simulink model "parcours_funktioniert"  (R2018a)
settings: Solver=ode1  StartTime=0.0  StopTime=inf  FixedStep=1/20  RelTol=1e-3  EnableMultiTasking=on
undefined symbols (not defined in the file): gray
libraries: simulink x6, visiontextngfix x4, visiontransforms x4, visionanalysis x2, visionstatistics x2, PiCar_library x1, embdlinuxlib x1
settings Model: SimulationMode=external  Creator=raspberry  LastModifiedBy=dave
settings SolverCC: PositivePriorityOrder=on
settings OptimizationCC: PassReuseOutputArgsAs=Individual arguments  MaxStackSize=64
settings DebuggingCC: ParameterTunabilityLossMsg=error
settings HardwareCC: ProdBitPerPointer=32  ProdBitPerSizeT=32  ProdBitPerPtrDiffT=32  ProdLargestAtomicInteger=Long  ProdLargestAtomicFloat=Double  ProdWordSize=32  ProdHWDeviceType=ARM Compatible->ARM Cortex
settings SFSimCC: MATLABDynamicMemAlloc=off
settings RTWCC: SystemTargetFile=ert.tlc  HardwareBoard=Raspberry Pi  TLCOptions="-aInlineSetEventsForThisBaseRateFcn=TLC_FALSE -aSuppressMultiTaskScheduler=TLC_FALSE  -aRateBasedStepFcn=0"  TemplateMakefile=ert_default_tmf  Toolchain=GNU GCC Raspberry Pi
settings RTWCC: CustomTerminator=|
  | /* Send ALL_LED_OFF Signal to all PWM driver chip address
  | See PCA9685 user manual, section 7.3.4
  | Set Chip in sleep mode, section 7.3.1
  | Reset the PWM ON/OFF states for all LEDs */
  | 
  | int fd;
  | 
  | fd = wiringPiI2CSetup(0x70);
  | wiringPiI2CWriteReg8(fd, 0x00, 0x11); // sleep mode
  | wiringPiI2CWriteReg8(fd, 0xFD, 0x10); // all LED off
  | wiringPiI2CWriteReg8(fd, 0xFC, 0x00);
  | wiringPiI2CWriteReg8(fd, 0xFB, 0x00);
  | wiringPiI2CWriteReg8(fd, 0xFA, 0x00);
settings CodeAppCC: ForceParamTrailComments=on  IgnoreCustomStorageClasses=off  OperatorAnnotations=on  SimulinkDataObjDesc=on  SFDataObjDesc=on  MATLABFcnDesc=on  InsertBlockDesc=on  StateflowObjectComments=on  MATLABSourceComments=on
settings ERTTargetCC: SupportVariableSizeSignals=on

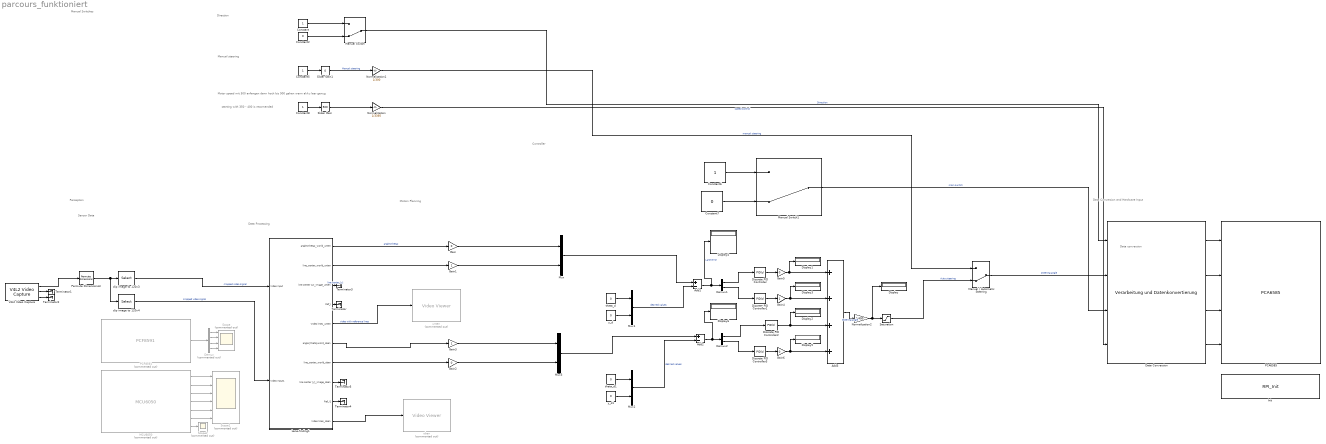
== system parcours_funktioniert ==
  note: starting with 350 - 400 is recomended
  note: Data Conversion and Hardware Input
  note: Data conversion
  note: Manual Switches
  note: Motion Planning
  note: Perception
  note: Controller
  note: Data Processing
  note: Sensor Data
  note: Manual steering
  note: Motor speed
      | mit 500 anfangen
      | dann hoch bis 900
      | gehen wenn akku
      | leer genug
  note: Direction
  Add1 : Sum  Inputs=+-
  Add2 : Sum  Inputs=+-
  Add3 : Sum  Inputs=++++
  Constant{,5..6,8} (4 alike) : Constant
  Constant2 : Constant  Value=0
  Constant7 : Constant  Value=0
  Data Conversion : PiCar_library/Verarbeitung und Datenkonvertierung
      link override Constant3: Value=1160
  Demux : Demux  Commented=on
  Demux1 : Demux  Outputs=2
  Demux2 : Demux  Outputs=2
  Discrete PID Controller : simulink/Continuous/PID Controller  Controller=PID  TimeDomain=Discrete-time  SampleTime=-1  IntegratorMethod=Forward Euler  FilterMethod=Forward Euler  Form=Parallel  UseFilter=on  ControllerParametersSource=internal  P=0  I=0  D=0  N=100  InitialConditionSource=internal  InitialConditionForIntegrator=0  InitialConditionForFilter=0  ExternalReset=none  LimitOutput=off  UpperSaturationLimit=inf  LowerSaturationLimit=-inf  LinearizeAsGain=off  AntiWindupMode=none  Kb=1  TrackingMode=off  Kt=1  PParamMin=[]  PParamMax=[]  IParamMin=[]  IParamMax=[]  DParamMin=[]  DParamMax=[]  NParamMin=[]  NParamMax=[]  KbParamMin=[]  KbParamMax=[]  KtParamMin=[]  KtParamMax=[]  POutMin=[]  POutMax=[]  IOutMin=[]  IOutMax=[]  DOutMin=[]  DOutMax=[]  NOutMin=[]  NOutMax=[]  KbOutMin=[]  KbOutMax=[]  KtOutMin=[]  KtOutMax=[]  IntegratorOutMin=[]  IntegratorOutMax=[]  FilterOutMin=[]  FilterOutMax=[]  SumOutMin=[]  SumOutMax=[]  SumI1OutMin=[]  SumI1OutMax=[]  SumI2OutMin=[]  SumI2OutMax=[]  SumI3OutMin=[]  SumI3OutMax=[]  SumDOutMin=[]  SumDOutMax=[]  SaturationOutMin=[]  SaturationOutMax=[]  IntegratorContinuousStateAttributes=''  IntegratorStateMustResolveToSignalObject=off  IntegratorRTWStateStorageClass=Auto  FilterContinuousStateAttributes=''  FilterStateMustResolveToSignalObject=off  FilterRTWStateStorageClass=Auto  DifferentiatorICPrevScaledInput=0  DifferentiatorOutMin=[]  DifferentiatorOutMax=[]  FilterDiffOutCoefMin=[]  FilterDiffOutCoefMax=[]  SumDenOutMin=[]  SumDenOutMax=[]  SumNumOutMin=[]  SumNumOutMax=[]  ReciprocalOutMin=[]  ReciprocalOutMax=[]  DivideOutMin=[]  DivideOutMax=[]  TunerSelectOption=Transfer Function Based (PID Tuner App)
  Discrete PID Controller1 : simulink/Continuous/PID Controller  Controller=PID  TimeDomain=Discrete-time  SampleTime=-1  IntegratorMethod=Forward Euler  FilterMethod=Forward Euler  Form=Parallel  UseFilter=on  ControllerParametersSource=internal  P=1  I=0  D=0  N=100  InitialConditionSource=internal  InitialConditionForIntegrator=0  InitialConditionForFilter=0  ExternalReset=none  LimitOutput=off  UpperSaturationLimit=inf  LowerSaturationLimit=-inf  LinearizeAsGain=off  AntiWindupMode=none  Kb=1  TrackingMode=off  Kt=1  PParamMin=[]  PParamMax=[]  IParamMin=[]  IParamMax=[]  DParamMin=[]  DParamMax=[]  NParamMin=[]  NParamMax=[]  KbParamMin=[]  KbParamMax=[]  KtParamMin=[]  KtParamMax=[]  POutMin=[]  POutMax=[]  IOutMin=[]  IOutMax=[]  DOutMin=[]  DOutMax=[]  NOutMin=[]  NOutMax=[]  KbOutMin=[]  KbOutMax=[]  KtOutMin=[]  KtOutMax=[]  IntegratorOutMin=[]  IntegratorOutMax=[]  FilterOutMin=[]  FilterOutMax=[]  SumOutMin=[]  SumOutMax=[]  SumI1OutMin=[]  SumI1OutMax=[]  SumI2OutMin=[]  SumI2OutMax=[]  SumI3OutMin=[]  SumI3OutMax=[]  SumDOutMin=[]  SumDOutMax=[]  SaturationOutMin=[]  SaturationOutMax=[]  IntegratorContinuousStateAttributes=''  IntegratorStateMustResolveToSignalObject=off  IntegratorRTWStateStorageClass=Auto  FilterContinuousStateAttributes=''  FilterStateMustResolveToSignalObject=off  FilterRTWStateStorageClass=Auto  DifferentiatorICPrevScaledInput=0  DifferentiatorOutMin=[]  DifferentiatorOutMax=[]  FilterDiffOutCoefMin=[]  FilterDiffOutCoefMax=[]  SumDenOutMin=[]  SumDenOutMax=[]  SumNumOutMin=[]  SumNumOutMax=[]  ReciprocalOutMin=[]  ReciprocalOutMax=[]  DivideOutMin=[]  DivideOutMax=[]  TunerSelectOption=Transfer Function Based (PID Tuner App)
  Discrete PID Controller2 : simulink/Continuous/PID Controller  Controller=PID  TimeDomain=Discrete-time  SampleTime=-1  IntegratorMethod=Forward Euler  FilterMethod=Forward Euler  Form=Parallel  UseFilter=on  ControllerParametersSource=internal  P=10  I=0  D=0  N=100  InitialConditionSource=internal  InitialConditionForIntegrator=0  InitialConditionForFilter=0  ExternalReset=none  LimitOutput=off  UpperSaturationLimit=inf  LowerSaturationLimit=-inf  LinearizeAsGain=off  AntiWindupMode=none  Kb=1  TrackingMode=off  Kt=1  PParamMin=[]  PParamMax=[]  IParamMin=[]  IParamMax=[]  DParamMin=[]  DParamMax=[]  NParamMin=[]  NParamMax=[]  KbParamMin=[]  KbParamMax=[]  KtParamMin=[]  KtParamMax=[]  POutMin=[]  POutMax=[]  IOutMin=[]  IOutMax=[]  DOutMin=[]  DOutMax=[]  NOutMin=[]  NOutMax=[]  KbOutMin=[]  KbOutMax=[]  KtOutMin=[]  KtOutMax=[]  IntegratorOutMin=[]  IntegratorOutMax=[]  FilterOutMin=[]  FilterOutMax=[]  SumOutMin=[]  SumOutMax=[]  SumI1OutMin=[]  SumI1OutMax=[]  SumI2OutMin=[]  SumI2OutMax=[]  SumI3OutMin=[]  SumI3OutMax=[]  SumDOutMin=[]  SumDOutMax=[]  SaturationOutMin=[]  SaturationOutMax=[]  IntegratorContinuousStateAttributes=''  IntegratorStateMustResolveToSignalObject=off  IntegratorRTWStateStorageClass=Auto  FilterContinuousStateAttributes=''  FilterStateMustResolveToSignalObject=off  FilterRTWStateStorageClass=Auto  DifferentiatorICPrevScaledInput=0  DifferentiatorOutMin=[]  DifferentiatorOutMax=[]  FilterDiffOutCoefMin=[]  FilterDiffOutCoefMax=[]  SumDenOutMin=[]  SumDenOutMax=[]  SumNumOutMin=[]  SumNumOutMax=[]  ReciprocalOutMin=[]  ReciprocalOutMax=[]  DivideOutMin=[]  DivideOutMax=[]  TunerSelectOption=Transfer Function Based (PID Tuner App)
  Discrete PID Controller3 : simulink/Continuous/PID Controller  Controller=PID  TimeDomain=Discrete-time  SampleTime=-1  IntegratorMethod=Forward Euler  FilterMethod=Forward Euler  Form=Parallel  UseFilter=on  ControllerParametersSource=internal  P=0  I=0  D=0  N=100  InitialConditionSource=internal  InitialConditionForIntegrator=0  InitialConditionForFilter=0  ExternalReset=none  LimitOutput=off  UpperSaturationLimit=inf  LowerSaturationLimit=-inf  LinearizeAsGain=off  AntiWindupMode=none  Kb=1  TrackingMode=off  Kt=1  PParamMin=[]  PParamMax=[]  IParamMin=[]  IParamMax=[]  DParamMin=[]  DParamMax=[]  NParamMin=[]  NParamMax=[]  KbParamMin=[]  KbParamMax=[]  KtParamMin=[]  KtParamMax=[]  POutMin=[]  POutMax=[]  IOutMin=[]  IOutMax=[]  DOutMin=[]  DOutMax=[]  NOutMin=[]  NOutMax=[]  KbOutMin=[]  KbOutMax=[]  KtOutMin=[]  KtOutMax=[]  IntegratorOutMin=[]  IntegratorOutMax=[]  FilterOutMin=[]  FilterOutMax=[]  SumOutMin=[]  SumOutMax=[]  SumI1OutMin=[]  SumI1OutMax=[]  SumI2OutMin=[]  SumI2OutMax=[]  SumI3OutMin=[]  SumI3OutMax=[]  SumDOutMin=[]  SumDOutMax=[]  SaturationOutMin=[]  SaturationOutMax=[]  IntegratorContinuousStateAttributes=''  IntegratorStateMustResolveToSignalObject=off  IntegratorRTWStateStorageClass=Auto  FilterContinuousStateAttributes=''  FilterStateMustResolveToSignalObject=off  FilterRTWStateStorageClass=Auto  DifferentiatorICPrevScaledInput=0  DifferentiatorOutMin=[]  DifferentiatorOutMax=[]  FilterDiffOutCoefMin=[]  FilterDiffOutCoefMax=[]  SumDenOutMin=[]  SumDenOutMax=[]  SumNumOutMin=[]  SumNumOutMax=[]  ReciprocalOutMin=[]  ReciprocalOutMax=[]  DivideOutMin=[]  DivideOutMax=[]  TunerSelectOption=Transfer Function Based (PID Tuner App)
  Display{,1..6} (7 alike) : Display
  Gain{,2,5..6} (4 alike) : Gain  Gain=0
  Gain1 : Gain
  Gain3 : Gain
  Gain4 : Gain
  Init : S-Function  Priority=1  InitFcn=try, set_param(gcb,'FunctionName','RPI_Init'), end  FunctionName=RPI_Init  SFunctionModules=RPI_Init_wrapper  SFunctionDeploymentMode=off  EnableBusSupport=off  mask(S-Function Builder){}
      mask help: Simulink:masks:SFunctionBuilder_MD
      mask init:
      | val = [[.9  0.75 0.75 1 1 .9 .9 1]',[1 1 0.75 0.75 .9 .9 1 .9]'];try , sys = get_param(gcb,'SfunBuilderFcnName');if isempty(sys), sys = get_param(gcb,'FunctionName'); end,catch, sys = get_param(gcb,'FunctionName'); end
      settings: CopyFcn=set_param(gcbh,'LinkStatus','none')  PreSaveFcn=try, set_param(gcb,'FunctionName','RPI_Init'), end  OpenFcn=sfunctionwizard(gcbh)
      mask Display:
      | plot(val(:,1),val(:,2))
      | disp(sys)
  Lane-finding1 : Subsystem  AncestorBlock=PiCar_library/Lane-finding
  MCU6050 : S-Function  Commented=on  InitFcn=try, set_param(gcb,'FunctionName','MCU6050'), end  FunctionName=MCU6050  SFunctionModules=MCU6050_wrapper  SFunctionDeploymentMode=off  EnableBusSupport=off  mask(S-Function Builder){}
      mask help: Simulink:masks:SFunctionBuilder_MD
      mask init: same as parcours_funktioniert/Init
      settings: CopyFcn=set_param(gcbh,'LinkStatus','none')  PreSaveFcn=try, set_param(gcb,'FunctionName','MCU6050'), end  OpenFcn=sfunctionwizard(gcbh)
      mask Display: plot(val(:,1),val(:,2)),disp(sys), port_label('output',1,'ax'), port_label('output',2,'ay'), port_label('output',3,'az'), port_label('output',4,'omx'), port_label('output',5,'omy'), port_label('output',6,'omz'), port_label('output',7,'temp')
  Manual / Automatic Steering : ManualSwitch  CurrentSetting=0
  Manual Switch : ManualSwitch  CurrentSetting=0
  Manual Switch1 : ManualSwitch  CurrentSetting=0
  Mux{,1..3} (4 alike) : Mux  Inputs=2
  Normalization : Gain  Gain=1/3395
  Normalization1 : Gain  Gain=1/300
  Normalization2 : Gain  Gain=1/400
  PCA6585 : S-Function  InitFcn=try, set_param(gcb,'FunctionName','PCA6585'), end  FunctionName=PCA6585  SFunctionModules=PCA6585_wrapper  SFunctionDeploymentMode=off  EnableBusSupport=off  mask(S-Function Builder){}
      mask help: Simulink:masks:SFunctionBuilder_MD
      mask init: same as parcours_funktioniert/Init
      settings: CopyFcn=set_param(gcbh,'LinkStatus','none')  PreSaveFcn=try, set_param(gcb,'FunctionName','PCA6585'), end  OpenFcn=sfunctionwizard(gcbh)
      mask Display: plot(val(:,1),val(:,2)),disp(sys), port_label('input',1,'IN_1'), port_label('input',2,'IN_2'), port_label('input',3,'PWM'), port_label('input',4,'SERVO')
  PCF8591 : S-Function  Commented=on  InitFcn=try, set_param(gcb,'FunctionName','PCF8591'), end  FunctionName=PCF8591  SFunctionModules=PCF8591_wrapper  SFunctionDeploymentMode=off  EnableBusSupport=off  mask(S-Function Builder){}
      mask help: Simulink:masks:SFunctionBuilder_MD
      mask init: same as parcours_funktioniert/Init
      settings: CopyFcn=set_param(gcbh,'LinkStatus','none')  PreSaveFcn=try, set_param(gcb,'FunctionName','PCF8591'), end  OpenFcn=sfunctionwizard(gcbh)
      mask Display: plot(val(:,1),val(:,2)),disp(sys), port_label('output',1,'PCF8591_out')
  Permute Dimensions3 : PermuteDimensions
  Saturation : Saturate  UpperLimit=1  LowerLimit=-1
  Scope : Scope  Commented=on  NumInputPorts=4
  Scope1 : Scope  Commented=on  NumInputPorts=6
  Scope2 : Scope  Commented=on
  Slider Gain : simulink/Math Operations/Slider Gain  gain=500  low=0  high=3395
  Slider Gain1 : simulink/Math Operations/Slider Gain  gain=0  low=-300  high=300
  Terminator{,1..5} (6 alike) : Terminator
  V4L2 Video Capture : embdlinuxlib/V4L2 Video Capture  m_devName='/dev/video0'  roi=[0, 0, 640, 480]  imSizeSelection=320x240  imSize=[640, 480]  pixelFormat=YCbCr 4:2:2  pixelOrder=Planar  sampleTime=1/20  simOutput=Colorbars  blockPlatform=Raspberry Pi
      settings: SourceProductName=Simulink Support Package for Raspberry Pi Hardware  SourceProductBaseCode=RASPPI
  clip image to 120x3 : Selector  NumberOfDimensions=2  InputPortWidth=3  IndexOptions=Index vector (dialog),Index vector (dialog)  Indices=[180:1:200],[1:4:320]  OutputSizes=1,1
  clip image to 120x4 : Selector  NumberOfDimensions=2  InputPortWidth=3  IndexOptions=Index vector (dialog),Index vector (dialog)  Indices=[120:1:180],[1:4:320]  OutputSizes=1,1
  oben : VideoViewer  Commented=on  colormapValue=gray(256)  FigPos=[37.8 442.8 582.4 304.8]
  theta_d : Constant  Value=0
  theta_d1 : Constant  Value=0
  unten : VideoViewer  Commented=on  colormapValue=gray(256)  FigPos=[19.4 847.6 603.2 284.8]
  y_d : Constant  Value=0
  y_d1 : Constant  Value=0
  wires:
  Constant/1 -> Manual Switch/1
  Constant2/1 -> Manual Switch/2
  Constant7/1 -> Manual Switch1/2
  Constant6/1 -> Manual Switch1/1
  Constant8/1 -> Slider Gain/1
  Slider Gain1/1 -> Normalization1/1  "Manual steering"
  Constant5/1 -> Slider Gain1/1
  Demux/3 -> Scope/3
  Demux/4 -> Scope/4
  PCF8591/1 -> Demux/1
  MCU6050/2 -> Scope1/2
  MCU6050/3 -> Scope1/3
  MCU6050/1 -> Scope1/1
  MCU6050/4 -> Scope1/4
  MCU6050/5 -> Scope1/5
  MCU6050/6 -> Scope1/6
  MCU6050/7 -> Scope2/1
  Manual Switch/1 -> Data Conversion/1  "Direction"
  Manual / Automatic Steering/1 -> Data Conversion/2  "steering angle"
  Manual Switch1/1 -> Data Conversion/3  "main switch"
  Data Conversion/1 -> PCA6585/1
  Data Conversion/2 -> PCA6585/2
  Data Conversion/3 -> PCA6585/3
  Data Conversion/4 -> PCA6585/4
  clip image to 120x3/1 -> Lane-finding1/1(Video input)  "cropped video signal"
  Lane-finding1/1(angle [theta]_world_unten) -> Gain/1  "angle [theta]"
  Slider Gain/1 -> Normalization/1
  Lane-finding1/4(Ref_I) -> Terminator/1
  Lane-finding1/5(Video lines_unten) -> unten/1  "video with reference lines"
  Normalization/1 -> Data Conversion/4  "speed control"
  y_d/1 -> Mux1/2
  theta_d/1 -> Mux1/1
  Mux1/1 -> Add1/2  "desired values"
  Normalization1/1 -> Manual / Automatic Steering/1  "manual steering"
  Demux/1 -> Scope/1
  Demux/2 -> Scope/2
  Permute Dimensions3/1 -> clip image to 120x4/1, clip image to 120x3/1
  V4L2 Video Capture/1 -> Permute Dimensions3/1
  V4L2 Video Capture/2 -> Terminator1/1
  V4L2 Video Capture/3 -> Terminator2/1
  clip image to 120x4/1 -> Lane-finding1/2(Video input1)  "cropped video signal"
  Lane-finding1/10(Video lines_oben) -> oben/1
  Discrete PID Controller/1 -> Gain5/1
  Add1/1 -> Display4/1, Demux1/1  "Lane error"
  Add3/1 -> Normalization2/1  "Steering angle"
  Saturation/1 -> Manual / Automatic Steering/2  "Auto steering"
  Normalization2/1 -> Display/1, Saturation/1
  Mux/1 -> Add1/1
  Discrete PID Controller1/1 -> Gain4/1
  Demux1/2 -> Discrete PID Controller1/1
  Demux1/1 -> Discrete PID Controller/1
  Discrete PID Controller2/1 -> Add3/3, Display2/1
  Discrete PID Controller3/1 -> Gain6/1
  y_d1/1 -> Mux2/2
  theta_d1/1 -> Mux2/1
  Mux2/1 -> Add2/2  "desired values"
  Lane-finding1/2(line_center_world_unten) -> Gain1/1
  Mux3/1 -> Add2/1
  Demux2/2 -> Discrete PID Controller3/1
  Add2/1 -> Display6/1, Demux2/1
  Lane-finding1/6(angle [theta]wolrd_oben) -> Gain3/1
  Gain/1 -> Mux/1
  Gain1/1 -> Mux/2
  Lane-finding1/3(line center [y]_image_unten) -> Terminator3/1  "line center [y]"
  Lane-finding1/7(line_center_world_oben) -> Gain2/1
  Gain2/1 -> Mux3/2
  Gain3/1 -> Mux3/1
  Lane-finding1/8(line center [y]_image_oben) -> Terminator5/1
  Lane-finding1/9(Ref_I1) -> Terminator4/1
  Gain4/1 -> Display3/1, Add3/2
  Gain5/1 -> Display1/1, Add3/1
  Gain6/1 -> Display5/1, Add3/4
  Demux2/1 -> Discrete PID Controller2/1

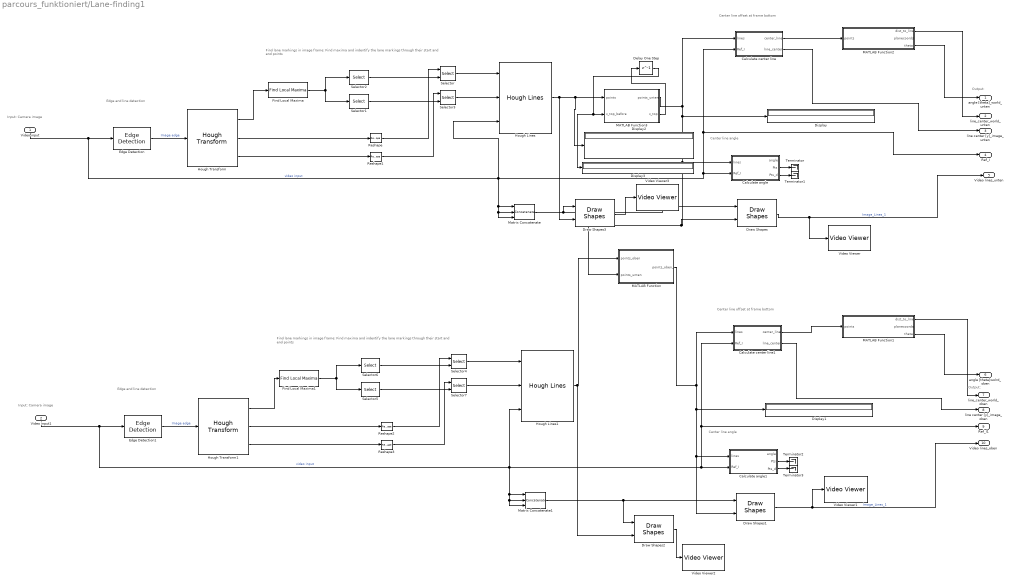
== system parcours_funktioniert/Lane-finding1 ==
  note: Output:
  note: Input: Camera image
  note: Edge and line detection
  note: Find lane markings in image frame:
      | Find maxima and indentify the lane markings through their start and end points
  note: Center line angle
  note: Center line offset at frame bottom
  note: Center line angle
  note: Output:
  note: Find lane markings in image frame:
      | Find maxima and indentify the lane markings through their start and end points
  note: Edge and line detection
  note: Input: Camera image
  note: Center line offset at frame bottom
  Video input : Inport
  Video input1 : Inport  Port=2
  Calculate angle : MATLAB Function  TreatAsAtomicUnit=on
  Calculate angle1 : MATLAB Function  TreatAsAtomicUnit=on
  Calculate center line : MATLAB Function  TreatAsAtomicUnit=on
  Calculate center line1 : MATLAB Function  TreatAsAtomicUnit=on
  Delay One Step : Delay  DelayLength=1
  Display{,1..3} (4 alike) : Display
  Draw Shapes{,1..3} (4 alike) : visiontextngfix/Draw Shapes  shape=Lines  fill=off  lineWidth=1  fillClrSource=Specify via dialog  display=User-specified value  intensity=200  color=[0 0 255]  opacity=0.6  viewport=Entire image  antialiasing=off  inType=Obsolete  imagePorts=One multidimensional signal  prodOutputMode=Binary point scaling  prodOutputWordLength=32  prodOutputFracLength=14  memoryMode=Specify word length  memoryWordLength=16  memoryFracLength=14  roundingMode=Floor  overflowMode=off
      settings: SourceProductName=Computer Vision System Toolbox
  Edge Detection : visionanalysis/Edge Detection  method=Sobel  outputType=Binary image  userDefinedThreshold=off  thresholdSource=Input port  threshold=20  thresholdTuning=4  edgeThinning=off  threshold_canny=[0.25 0.60]  autoPercent=70  sigma=1  roundingMode=Floor  overflowMode=off  prodOutputMode=Binary point scaling  prodOutputWordLength=32  prodOutputFracLength=8  prodOutputSlope=2^-8  accumSlope=2^-8  outputSlope=2^-4
      settings: SourceProductName=Computer Vision System Toolbox  SourceProductBaseCode=VP
  Edge Detection1 : visionanalysis/Edge Detection  method=Sobel  outputType=Binary image  userDefinedThreshold=off  thresholdSource=Input port  threshold=20  thresholdTuning=4  edgeThinning=off  threshold_canny=[0.25 0.60]  autoPercent=70  sigma=1  roundingMode=Floor  overflowMode=off  prodOutputMode=Binary point scaling  prodOutputWordLength=32  prodOutputFracLength=8  prodOutputSlope=2^-8  accumSlope=2^-8  outputSlope=2^-4
      settings: SourceProductName=Computer Vision System Toolbox  SourceProductBaseCode=VP
  Find Local Maxima : visionstatistics/Find Local Maxima  num_peaks=6  nhood_size=[5 7]  src_thresh=Obsolete9b  src_thresh_inuse=Specify via dialog  threshold=10  inputIsHough=off  dt_peak=uint32  isOutVarDim=on  dt_count=uint32
      settings: SourceProductName=Computer Vision System Toolbox  SourceProductBaseCode=VP
  Find Local Maxima1 : visionstatistics/Find Local Maxima  num_peaks=16  nhood_size=[5 7]  src_thresh=Obsolete9b  src_thresh_inuse=Specify via dialog  threshold=10  inputIsHough=off  dt_peak=uint32  isOutVarDim=on  dt_count=uint32
      settings: SourceProductName=Computer Vision System Toolbox  SourceProductBaseCode=VP
  Hough Lines : visiontransforms/Hough Lines  sineCompMethod=Trigonometric function  thetaRes=pi/180  firstCoeffMode=Specify word length  firstCoeffWordLength=16  firstCoeffFracLength=15  prodOutputMode=Binary point scaling  prodOutputWordLength=32  prodOutputFracLength=16  roundingMode=Nearest  overflowMode=on
      settings: SourceProductName=Computer Vision System Toolbox  SourceProductBaseCode=VP
  Hough Lines1 : visiontransforms/Hough Lines  sineCompMethod=Trigonometric function  thetaRes=pi/180  firstCoeffMode=Specify word length  firstCoeffWordLength=16  firstCoeffFracLength=15  prodOutputMode=Binary point scaling  prodOutputWordLength=32  prodOutputFracLength=16  roundingMode=Nearest  overflowMode=on
      settings: SourceProductName=Computer Vision System Toolbox  SourceProductBaseCode=VP
  Hough Transform : visiontransforms/Hough Transform  theta_res=pi/180  rho_res=1  out_theta_rho=on  outdtmode=double  firstCoeffMode=Binary point scaling  firstCoeffWordLength=16  firstCoeffFracLength=14  secondCoeffMode=Binary point scaling  secondCoeffWordLength=32  secondCoeffFracLength=16  outputMode=Binary point scaling  outputWordLength=16  outputFracLength=0  accumMode=Binary point scaling  accumWordLength=32  accumFracLength=20  prodOutputMode=Binary point scaling  prodOutputWordLength=32  prodOutputFracLength=20  memoryMode=Binary point scaling  memoryWordLength=32  memoryFracLength=16  roundingMode=Nearest  overflowMode=on
      settings: SourceProductName=Computer Vision System Toolbox  SourceProductBaseCode=VP
  Hough Transform1 : visiontransforms/Hough Transform  theta_res=pi/180  rho_res=1  out_theta_rho=on  outdtmode=double  firstCoeffMode=Binary point scaling  firstCoeffWordLength=16  firstCoeffFracLength=14  secondCoeffMode=Binary point scaling  secondCoeffWordLength=32  secondCoeffFracLength=16  outputMode=Binary point scaling  outputWordLength=16  outputFracLength=0  accumMode=Binary point scaling  accumWordLength=32  accumFracLength=20  prodOutputMode=Binary point scaling  prodOutputWordLength=32  prodOutputFracLength=20  memoryMode=Binary point scaling  memoryWordLength=32  memoryFracLength=16  roundingMode=Nearest  overflowMode=on
      settings: SourceProductName=Computer Vision System Toolbox  SourceProductBaseCode=VP
  MATLAB Function : MATLAB Function  TreatAsAtomicUnit=on
  MATLAB Function1 : MATLAB Function  TreatAsAtomicUnit=on
  MATLAB Function2 : MATLAB Function  TreatAsAtomicUnit=on
  MATLAB Function3 : MATLAB Function  TreatAsAtomicUnit=on
  Matrix Concatenate : Concatenate  NumInputs=3  Mode=Multidimensional array  ConcatenateDimension=3
  Matrix Concatenate1 : Concatenate  NumInputs=3  Mode=Multidimensional array  ConcatenateDimension=3
  Reshape{,1..3} (4 alike) : Reshape
  Selector{,3..4,7} (4 alike) : Selector  IndexOptions=Index vector (port)  Indices=[1 3]  OutputSizes=1
  Selector1 : Selector  NumberOfDimensions=2  InputPortWidth=3  IndexOptions=Select all,Index vector (dialog)  Indices=[1 3],2  OutputSizes=1,1
  Selector2 : Selector  NumberOfDimensions=2  InputPortWidth=3  IndexOptions=Select all,Index vector (dialog)  Indices=[1 3],1  OutputSizes=1,1
  Selector5 : Selector  NumberOfDimensions=2  InputPortWidth=3  IndexOptions=Select all,Index vector (dialog)  Indices=[1 3],2  OutputSizes=1,1
  Selector6 : Selector  NumberOfDimensions=2  InputPortWidth=3  IndexOptions=Select all,Index vector (dialog)  Indices=[1 3],1  OutputSizes=1,1
  Terminator{,1..3} (4 alike) : Terminator
  Video Viewer : VideoViewer  colormapValue=gray(256)  FigPos=[153 1061 418 304]
  Video Viewer1 : VideoViewer  colormapValue=gray(256)  FigPos=[467 482 418 304]
  Video Viewer2 : VideoViewer  colormapValue=gray(256)  FigPos=[25 504 418 304]
  Video Viewer3 : VideoViewer  colormapValue=gray(256)  FigPos=[597 1007 408 304]
  angle [theta]_world_unten : Outport
  line_center_world_unten : Outport  Port=2
  line center [y]_image_unten : Outport  Port=3
  Ref_I : Outport  Port=4
  Video lines_unten : Outport  Port=5
  angle [theta]wolrd_oben : Outport  Port=6
  line_center_world_oben : Outport  Port=7
  line center [y]_image_oben : Outport  Port=8
  Ref_I1 : Outport  Port=9
  Video lines_oben : Outport  Port=10
  wires:
  MATLAB Function3/1(points_unten) -> MATLAB Function/2(points_unten), Draw Shapes/2, Calculate angle/1(lines), Display/1, Calculate center line/1(lines)
  Draw Shapes/1 -> Video Viewer/1, Video lines_unten/1  "Image_Lines_1"
  Matrix Concatenate/1 -> Draw Shapes3/1, Draw Shapes/1
  Reshape1/1 -> Selector3/1
  Selector3/1 -> Hough Lines/2
  Reshape/1 -> Selector/1
  Selector/1 -> Hough Lines/1
  Find Local Maxima/1 -> Selector1/1, Selector2/1
  Selector2/1 -> Selector/2
  Selector1/1 -> Selector3/2
  Hough Transform/1 -> Find Local Maxima/1
  Hough Transform/3 -> Reshape1/1
  Hough Transform/2 -> Reshape/1
  Video input/1 -> Edge Detection/1, Matrix Concatenate/3, Matrix Concatenate/2, Matrix Concatenate/1, Hough Lines/3, Calculate center line/2(Ref_I), Ref_I/1, Calculate angle/2(Ref_I)  "video input"
  Edge Detection/1 -> Hough Transform/1  "Image edge"
  Calculate angle/3(Pts_d) -> Terminator1/1
  Calculate angle/2(Pts) -> Terminator/1
  Selector5/1 -> Selector7/2
  Selector4/1 -> Hough Lines1/1
  Reshape2/1 -> Selector4/1
  Draw Shapes1/1 -> Video Viewer1/1, Video lines_oben/1  "Image_Lines_1"
  Edge Detection1/1 -> Hough Transform1/1  "Image edge"
  Matrix Concatenate1/1 -> Draw Shapes2/1, Draw Shapes1/1
  Calculate angle1/2(Pts) -> Terminator2/1
  Find Local Maxima1/1 -> Selector5/1, Selector6/1
  Calculate angle1/3(Pts_d) -> Terminator3/1
  Selector6/1 -> Selector4/2
  Video input1/1 -> Edge Detection1/1, Matrix Concatenate1/3, Matrix Concatenate1/2, Matrix Concatenate1/1, Hough Lines1/3, Calculate center line1/2(Ref_I), Ref_I1/1, Calculate angle1/2(Ref_I)  "video input"
  Hough Transform1/3 -> Reshape3/1
  MATLAB Function/1(points_oben_) -> Calculate center line1/1(lines), Calculate angle1/1(lines), Draw Shapes1/2, Display1/1
  Selector7/1 -> Hough Lines1/2
  Hough Transform1/1 -> Find Local Maxima1/1
  Reshape3/1 -> Selector7/1
  Hough Transform1/2 -> Reshape2/1
  Hough Lines1/1 -> Draw Shapes2/2, MATLAB Function/1(points_oben)
  Calculate center line/1(center_line) -> MATLAB Function2/1(points)
  Calculate center line/2(line_center) -> line center [y]_image_unten/1
  MATLAB Function2/3(theta) -> angle [theta]_world_unten/1
  Calculate center line1/1(center_line) -> MATLAB Function1/1(points)
  MATLAB Function1/3(theta) -> angle [theta]wolrd_oben/1
  Calculate center line1/2(line_center) -> line center [y]_image_oben/1
  MATLAB Function1/1(dist_to_line) -> line_center_world_oben/1
  MATLAB Function2/1(dist_to_line) -> line_center_world_unten/1
  Delay One Step/1 -> MATLAB Function3/2(x_top_before), Display3/1
  Draw Shapes2/1 -> Video Viewer2/1
  MATLAB Function3/2(x_top) -> Delay One Step/1
  Hough Lines/1 -> Draw Shapes3/2, Display2/1, MATLAB Function3/1(points)
  Draw Shapes3/1 -> Video Viewer3/1

== matlab function parcours_funktioniert/Lane-finding1/MATLAB Function ==
  data: points_oben input; points_oben_ output; points_unten input
function points_oben_  = chooseLine(points_oben, points_unten)
 points_oben_2 = zeros(2,4);
 n = size(points_oben,1);
 dist = zeros(n);
 
 for j = 1:1:2
     for i = 1:1:n
         dist(i) = abs(points_oben(i,3)-points_unten(j,1));
     end
     [~,I] = min(dist);
 
     for k = 1:1:4
         points_oben_2(j,k) = points_oben(I(1),k); 
     end
 end
 
 
 points_oben_ = int32(points_oben_2);
 end

== matlab function parcours_funktioniert/Lane-finding1/Calculate center line ==
  data: center_line output; line_center output; lines input; Ref_I input
function [center_line, line_center] = center(lines, Ref_I)

IMAGE_SIZE = size(Ref_I);
IMAGE_HEIGHT = IMAGE_SIZE(1);
IMAGE_WIDTH = IMAGE_SIZE(2);
points = zeros(2,4);

% Sorting the lines
if double(lines(1,1)) < double(lines(2,1))
    points(1,:) = lines(1,:);
    points(2,:) = lines(2,:);
else
    points(1,:) = lines(2,:);
    points(2,:) = lines(1,:);
end

% Calculate the lane center, top and bottom
x_center = double((points(1,:) + points(2,:))/2);

% Output the lane center at the bottom of the picture
line_center = x_center(3);
center_line = x_center;

== matlab function parcours_funktioniert/Lane-finding1/Calculate angle ==
  data: lines input; angle output; Pts output; Pts_d output; Ref_I input
function [angle, Pts, Pts_d] = angle(lines, Ref_I)

IMAGE_SIZE = size(Ref_I);
IMAGE_HEIGHT = IMAGE_SIZE(1);
IMAGE_WIDTH = IMAGE_SIZE(2);
points = zeros(2,4);

% Sorting the lines
if double(lines(1,1)) < double(lines(2,1))
    points(1,:) = lines(1,:);
    points(2,:) = lines(2,:);
else
    points(1,:) = lines(2,:);
    points(2,:) = lines(1,:);
end

% Calculate the lane center, top and bottom
x_center = double((points(1,:) + points(2,:))/2);

% Calculate the angle of the centerline: 0 -> vertical
angle = atan((x_center(3) - x_center(1))/IMAGE_HEIGHT);

% Auxilliary lines
Pts = int32([x_center(1), 1, x_center(3), 75]);
Pts_d = int32([IMAGE_WIDTH/2, 1, IMAGE_WIDTH/2, 75]);

% angles = atan2d(double((lines(:,1) - lines(:,3))), -double(lines(:,2) - lines(:,4)));

== matlab function parcours_funktioniert/Lane-finding1/Calculate angle1 ==
  data: lines input; angle output; Pts output; Pts_d output; Ref_I input
function [angle, Pts, Pts_d] = angle(lines, Ref_I)

IMAGE_SIZE = size(Ref_I);
IMAGE_HEIGHT = IMAGE_SIZE(1);
IMAGE_WIDTH = IMAGE_SIZE(2);
points = zeros(2,4);

% Sorting the lines
if double(lines(1,1)) < double(lines(2,1))
    points(1,:) = lines(1,:);
    points(2,:) = lines(2,:);
else
    points(1,:) = lines(2,:);
    points(2,:) = lines(1,:);
end

% Calculate the lane center, top and bottom
x_center = double((points(1,:) + points(2,:))/2);

% Calculate the angle of the centerline: 0 -> vertical
angle = atan((x_center(3) - x_center(1))/IMAGE_HEIGHT);

% Auxilliary lines
Pts = int32([x_center(1), 1, x_center(3), 75]);
Pts_d = int32([IMAGE_WIDTH/2, 1, IMAGE_WIDTH/2, 75]);

% angles = atan2d(double((lines(:,1) - lines(:,3))), -double(lines(:,2) - lines(:,4)));

== matlab function parcours_funktioniert/Lane-finding1/Calculate center line1 ==
  data: center_line output; line_center output; lines input; Ref_I input
function [center_line, line_center] = center(lines, Ref_I)

IMAGE_SIZE = size(Ref_I);
IMAGE_HEIGHT = IMAGE_SIZE(1);
IMAGE_WIDTH = IMAGE_SIZE(2);
points = zeros(2,4);

% Sorting the lines
if double(lines(1,1)) < double(lines(2,1))
    points(1,:) = lines(1,:);
    points(2,:) = lines(2,:);
else
    points(1,:) = lines(2,:);
    points(2,:) = lines(1,:);
end

% Calculate the lane center, top and bottom
x_center = double((points(1,:) + points(2,:))/2);

% Output the lane center at the bottom of the picture
line_center = x_center(3);
center_line = x_center;

== matlab function parcours_funktioniert/Lane-finding1/MATLAB Function1 ==
  data: dist_to_line output; planecoords output; theta output; points input
function [dist_to_line, planecoords, theta]  = CamToWorld(points)

pixelcoords = zeros(2,2);
pixelcoords(1,:) = points(1,1:2);
pixelcoords(2,:) = points(1,3:4);


pos = zeros(2,3);

for i = 1:1:2
    pixelcoord = pixelcoords(i,:);
    pixelcoord(1) = pixelcoord(1) * 4;
    pixelcoord(2) =  pixelcoord(2) * 1 + 120;
    plane_height = 0;  %77 bei Iske Buch
    alpha = 18.5; %18.5
    h= 275 - plane_height;
    f_px =[276.3065;275.7723];
    image_size = [320;240];
    camera_pos = [0;275;-315];

    %Pixelkoordinatensystem verschieben
    pixelcoord(1) = pixelcoord(1) - image_size(1)/2;
    pixelcoord(2) = -pixelcoord(2) + image_size(2)/2;

    %Position sch?tzen
    alpha = alpha * pi / 180;
    z_est = h/cos(alpha) / (tan(alpha) - pixelcoord(2)/f_px(2));
    y_est = z_est * pixelcoord(2)/f_px(2);
    x_est = z_est * pixelcoord(1)/f_px(1);

    %rotieren
    pos1 = [1 0 0; 0 cos(alpha) -sin(alpha); 0 sin(alpha) cos(alpha)] * [x_est; y_est; z_est];

    %Position der Kamera einbeziehen
    pos(i,:) = pos1 + camera_pos; 
    
end

planecoords = zeros(2,2);
planecoords = pos(:,1:2:3);

x_diff = planecoords(2,1) - planecoords(1,1);
y_diff = planecoords(2,2) - planecoords(1,2);

theta = 0;
theta = atan(abs( x_diff / y_diff));
theta = theta * sign(planecoords(1,1));
theta = theta *180 / pi;

dist_to_line = planecoords(1,1);

== matlab function parcours_funktioniert/Lane-finding1/MATLAB Function2 ==
  data: dist_to_line output; planecoords output; theta output; points input
function [dist_to_line, planecoords, theta]  = CamToWorld(points)

pixelcoords = zeros(2,2);
pixelcoords(1,:) = points(1,1:2);
pixelcoords(2,:) = points(1,3:4);


pos = zeros(2,3);

for i = 1:1:2
    pixelcoord = pixelcoords(i,:);
    pixelcoord(1) = pixelcoord(1) * 4;
    pixelcoord(2) =  pixelcoord(2) * 1 + 190;
    plane_height = 0;  %77 bei Iske Buch
    alpha = 18.5; %18.5
    h= 275 - plane_height;
    f_px =[276.3065;275.7723];
    image_size = [320;240];
    camera_pos = [0;275;-315];

    %Pixelkoordinatensystem verschieben
    pixelcoord(1) = pixelcoord(1) - image_size(1)/2;
    pixelcoord(2) = -pixelcoord(2) + image_size(2)/2;

    %Position sch?tzen
    alpha = alpha * pi / 180;
    z_est = h/cos(alpha) / (tan(alpha) - pixelcoord(2)/f_px(2));
    y_est = z_est * pixelcoord(2)/f_px(2);
    x_est = z_est * pixelcoord(1)/f_px(1);

    %rotieren
    pos1 = [1 0 0; 0 cos(alpha) -sin(alpha); 0 sin(alpha) cos(alpha)] * [x_est; y_est; z_est];

    %Position der Kamera einbeziehen
    pos(i,:) = pos1 + camera_pos; 
    
end

planecoords = zeros(2,2);
planecoords = pos(:,1:2:3);

x_diff = planecoords(2,1) - planecoords(1,1);
y_diff = planecoords(2,2) - planecoords(1,2);

theta = 0;
theta = atan(abs( x_diff / y_diff));
theta = theta * sign(planecoords(1,1));
theta = theta *180 / pi;

dist_to_line = planecoords(1,1);

== matlab function parcours_funktioniert/Lane-finding1/MATLAB Function3 ==
  data: points input; points_unten output; x_top_before input; x_top output
function [points_unten, x_top] = chooseLine(points, x_top_before)
points_2 = zeros(2,4);
 n = size(points,1);
 dist = zeros(n);
 helper = -1;
 
 for j = 1:1:2
     for i = 1:1:n
         if (helper == i) 
             dist(i) = Inf;
         else
             dist(i) = abs(points(i,1)-x_top_before(j));
         end
     end
     [~,I] = min(dist);
     helper = I(1);
 
     for k = 1:1:4
         points_2(j,k) = points(I(1),k); 
     end
 end
 
 x_top = [points_2(1, 3), points_2(2, 3)];
 points_unten = int32(points_2);

%  points_unten_help = zeros(2,4);
%  n = size(points,1);
%  dist = zeros(n);
%  for i = 1:1:n
%      dist(i) = points(i,1)-center_line(1,1);
%  end
%  
% %  a1 = points(dist>=0);
% %  a2 = points(dist<=0);
%  [~,I1] = min(dist(dist>=0));
%  [~,I2] = min(abs(dist(dist<=0)));
%  
%  for k = 1:1:4
%      points_unten_help(1,k) = points(I1(1),k);
%      points_unten_help(2,k) = points(I2(1),k);
%      
%  end
%  
%  points_unten = int32(points_unten_help);
 end
